simulink model "lookupTableDynamic_TestGen34"  (R2017b)
settings: Solver=FixedStepDiscrete  StartTime=0.0  StopTime=10.0  RelTol=1e-3
libraries: simulink x1
settings Model: Creator=ktrinh  LastModifiedBy=ktrinh
settings DebuggingCC: ParameterOverflowMsg=none

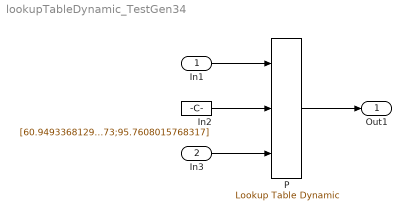
== system lookupTableDynamic_TestGen34 ==
  In1 : Inport  OutMin=58.9493  OutMax=97.7608  OutDataTypeStr=single  PortDimensions=3
  In3 : Inport  Port=2  PortDimensions=5
  In2 : Constant  Value=[60.9493368129351;81.8601982397284;86.6749981181823;90.4166615708573;95.7608015768317]  OutDataTypeStr=single
  P : simulink/Lookup Tables/Lookup Table Dynamic  LookUpMeth=Use Input Above  OutDataType=fixdt('int32')  OutScaling=[]  OutputDataTypeScalingMode=Specify via dialog  OutDataTypeStr=int32  RndMeth=Zero  DoSatur=off
      settings: SourceProductName=Simulink
  Out1 : Outport
  wires:
  In1/1 -> P/1
  In2/1 -> P/2
  In3/1 -> P/3
  P/1 -> Out1/1
